simulink model "timedIzhikevichTest"  (R2020b)
settings: Solver=VariableStepAuto  StartTime=0.0  StopTime=5000  FixedStep=0.001  RelTol=1e-3
libraries: simulink x2, dspsigops x1
settings Model: PacingRate=0.071000  Creator=40129232  LastModifiedBy=adamalcorn
settings SolverCC: AlgebraicLoopSolver=LineSearch
settings DataIOCC: ReturnWorkspaceOutputs=off
settings OptimizationCC: LifeSpan=inf
settings DebuggingCC: SFExecutionAtInitializationDiag=none  ArithmeticOperatorsInVariantConditions=warning
settings SFSimCC: SimUseLocalCustomCode=off  CustomCodeUndefinedFunction=UseInterfaceOnly
settings RTWCC: RTWUseLocalCustomCode=off
settings CodeAppCC: StateflowObjectComments=on

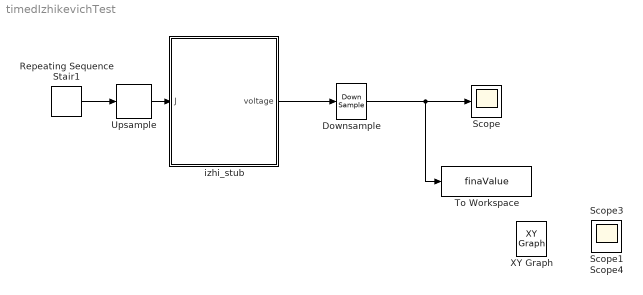
== system timedIzhikevichTest ==
  Downsample : DownSample  N=10  RateOptions=Allow multirate processing
  Repeating Sequence Stair1 : simulink/Sources/Repeating Sequence Stair  OutValues=[40.37, 52.35, 62.17, 70.19, 76.75].'  tsamp=10  OutMin=[]  OutMax=[]  OutDataTypeStr=double  OutputDataTypeScalingMode=double  OutDataType=fixdt(0,8)  ConRadixGroup=Best Precision: Vector-wise  OutScaling=2^-12
  Scope{,1,3..4} (4 alike) : Scope
  To Workspace : ToWorkspace  VariableName=finaValue  SaveFormat=Timeseries  SampleTime=-1
  Upsample : dspsigops/Upsample  N=10  phase=0  RateOptions=Allow multirate processing  ic=0  mode=Unused parameter value
  izhi_stub : Subsystem
  XY Graph : simulink/Sinks/XY Graph  IOType=viewer  xmin=-1  xmax=1  ymin=-1  ymax=1  st=-1
  wires:
  Repeating Sequence Stair1/1 -> Upsample/1
  Upsample/1 -> izhi_stub/1(J)
  Downsample/1 -> To Workspace/1, Scope/1
  izhi_stub/1(voltage) -> Downsample/1

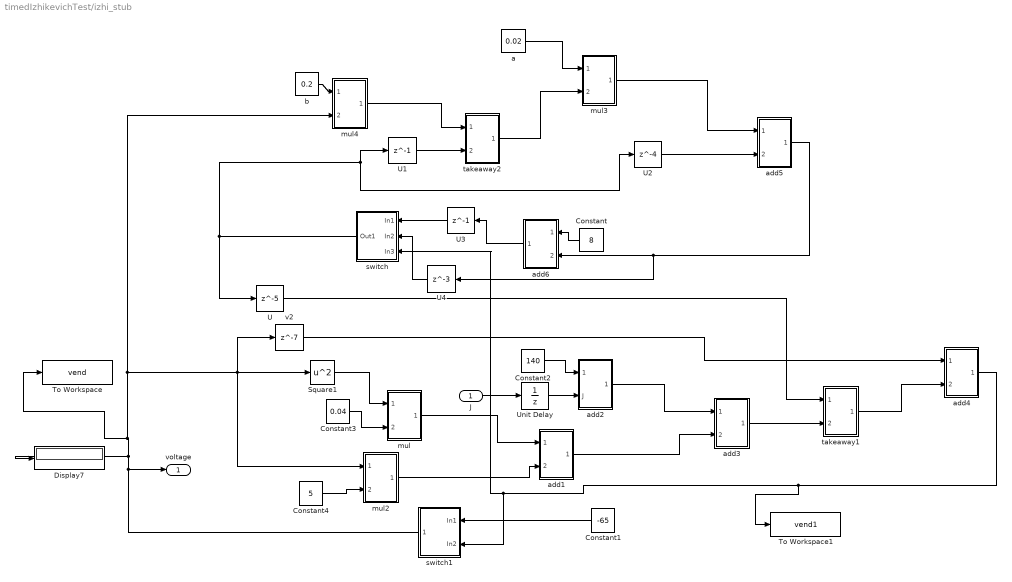
== system timedIzhikevichTest/izhi_stub ==
  J : Inport
  Constant : Constant  Value=8
  Constant1 : Constant  Value=-65
  Constant2 : Constant  Value=140
  Constant3 : Constant  Value=0.04
  Constant4 : Constant  Value=5
  Display7 : Display
  Square1 : Math  Operator=square  SaturateOnIntegerOverflow=on
  To Workspace : ToWorkspace  VariableName=vend  SaveFormat=Timeseries  SampleTime=-1
  To Workspace1 : ToWorkspace  VariableName=vend1  SaveFormat=Timeseries  SampleTime=-1
  U : Delay  DelayLength=5  InitialCondition=-65
  U1 : Delay  DelayLength=1  InitialCondition=0
  U2 : Delay  DelayLength=4  InitialCondition=0
  U3 : Delay  DelayLength=1  InitialCondition=0
  U4 : Delay  DelayLength=3  InitialCondition=0
  Unit Delay : UnitDelay  InitialCondition=-65  SampleTime=-1  HasFrameUpgradeWarning=on
  a : Constant  Value=0.02
  add1 : Subsystem
  add2 : Subsystem
  add3 : Subsystem
  add4 : Subsystem
  add5 : Subsystem
  add6 : Subsystem
  b : Constant  Value=0.2
  mul : Subsystem
  mul2 : Subsystem
  mul3 : Subsystem
  mul4 : Subsystem
  switch : Subsystem
  switch1 : Subsystem
  takeaway1 : Subsystem
  takeaway2 : Subsystem
  v2 : Delay  DelayLength=7  InitialCondition=-65
  voltage : Outport  VectorParamsAs1DForOutWhenUnconnected=off
  wires:
  Square1/1 -> mul/1(In1)
  Constant3/1 -> mul/2(In2)
  Constant4/1 -> mul2/2(In2)
  Constant2/1 -> add2/1(In1)
  Constant/1 -> add6/1(In1)
  a/1 -> mul3/1(In1)
  b/1 -> mul4/1(In1)
  Constant1/1 -> switch1/1(In1)
  add6/1(Out1) -> U3/1
  v2/1 -> add4/1(voltage)
  mul2/1(Out1) -> add1/2(In2)
  mul/1(Out1) -> add1/1(In1)
  add1/1(Out1) -> add3/2(In2)
  add3/1(Out1) -> takeaway1/2(In2)
  takeaway1/1(Out1) -> add4/2(In2)
  U/1 -> takeaway1/1(In1)
  add4/1(Out1) -> To Workspace1/1, switch/3(In3), switch1/2(In2)
  mul4/1(Out1) -> takeaway2/1(In1)
  switch/1(Out1) -> U1/1, U2/1, U/1
  U1/1 -> takeaway2/2(In2)
  U2/1 -> add5/2(In2)
  takeaway2/1(Out1) -> mul3/2(In2)
  mul3/1(Out1) -> add5/1(In1)
  add5/1(Out1) -> add6/2(In2), U4/1
  U4/1 -> switch/2(In2)
  U3/1 -> switch/1(In1)
  switch1/1(voltage) -> To Workspace/1, Square1/1, mul2/1(voltage), v2/1, mul4/2(voltage), Display7/1, voltage/1
  add2/1(Out1) -> add3/1(In1)
  J/1 -> Unit Delay/1
  Unit Delay/1 -> add2/2(J)

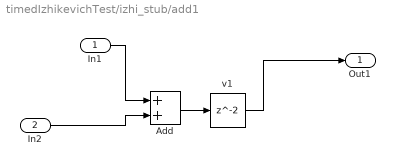
== system timedIzhikevichTest/izhi_stub/add1 ==
  In1 : Inport
  In2 : Inport  Port=2
  Add : Sum
  v1 : Delay  InitialCondition=-65
  Out1 : Outport
  wires:
  In2/1 -> Add/2
  In1/1 -> Add/1
  Add/1 -> v1/1
  v1/1 -> Out1/1

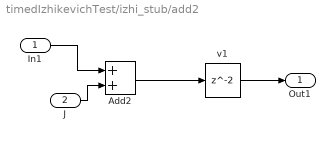
== system timedIzhikevichTest/izhi_stub/add2 ==
  In1 : Inport
  J : Inport  Port=2
  Add2 : Sum
  v1 : Delay  InitialCondition=-65
  Out1 : Outport
  wires:
  J/1 -> Add2/2
  In1/1 -> Add2/1
  Add2/1 -> v1/1
  v1/1 -> Out1/1

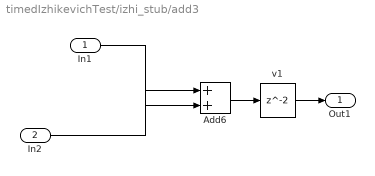
== system timedIzhikevichTest/izhi_stub/add3 ==
  In1 : Inport
  In2 : Inport  Port=2
  Add6 : Sum
  v1 : Delay  InitialCondition=-65
  Out1 : Outport
  wires:
  In2/1 -> Add6/1
  In1/1 -> Add6/2
  Add6/1 -> v1/1
  v1/1 -> Out1/1

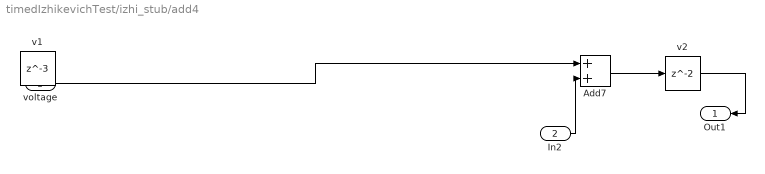
== system timedIzhikevichTest/izhi_stub/add4 ==
  voltage : Inport
  In2 : Inport  Port=2
  Add7 : Sum
  v1 : Delay  DelayLength=3  InitialCondition=0
  v2 : Delay  InitialCondition=-65
  Out1 : Outport
  wires:
  voltage/1 -> Add7/1
  In2/1 -> Add7/2
  Add7/1 -> v2/1
  v2/1 -> Out1/1

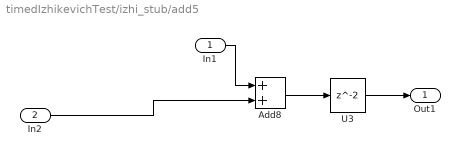
== system timedIzhikevichTest/izhi_stub/add5 ==
  In1 : Inport
  In2 : Inport  Port=2
  Add8 : Sum
  U3 : Delay  InitialCondition=0
  Out1 : Outport
  wires:
  In2/1 -> Add8/2
  In1/1 -> Add8/1
  Add8/1 -> U3/1
  U3/1 -> Out1/1

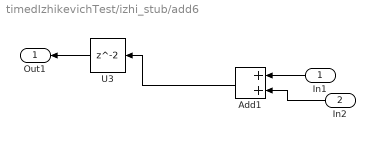
== system timedIzhikevichTest/izhi_stub/add6 ==
  In1 : Inport
  In2 : Inport  Port=2
  Add1 : Sum
  U3 : Delay  InitialCondition=0
  Out1 : Outport
  wires:
  In1/1 -> Add1/1
  In2/1 -> Add1/2
  Add1/1 -> U3/1
  U3/1 -> Out1/1

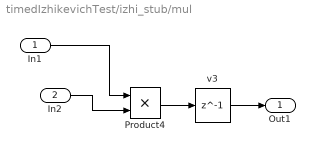
== system timedIzhikevichTest/izhi_stub/mul ==
  In1 : Inport
  In2 : Inport  Port=2
  Product4 : Product
  v3 : Delay  DelayLength=1  InitialCondition=-65
  Out1 : Outport
  wires:
  In2/1 -> Product4/2
  In1/1 -> Product4/1
  Product4/1 -> v3/1
  v3/1 -> Out1/1

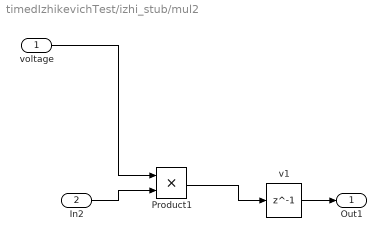
== system timedIzhikevichTest/izhi_stub/mul2 ==
  voltage : Inport
  In2 : Inport  Port=2
  Product1 : Product
  v1 : Delay  DelayLength=1  InitialCondition=-65
  Out1 : Outport
  wires:
  In2/1 -> Product1/2
  voltage/1 -> Product1/1
  Product1/1 -> v1/1
  v1/1 -> Out1/1

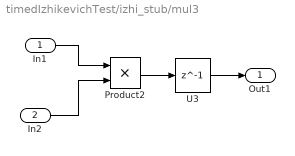
== system timedIzhikevichTest/izhi_stub/mul3 ==
  In1 : Inport
  In2 : Inport  Port=2
  Product2 : Product
  U3 : Delay  DelayLength=1  InitialCondition=0
  Out1 : Outport
  wires:
  In2/1 -> Product2/2
  In1/1 -> Product2/1
  Product2/1 -> U3/1
  U3/1 -> Out1/1

== system timedIzhikevichTest/izhi_stub/mul4 ==
  In1 : Inport
  voltage : Inport  Port=2
  Product3 : Product
  U2 : Delay  DelayLength=1  InitialCondition=0
  Out1 : Outport
  wires:
  voltage/1 -> Product3/2
  In1/1 -> Product3/1
  Product3/1 -> U2/1
  U2/1 -> Out1/1

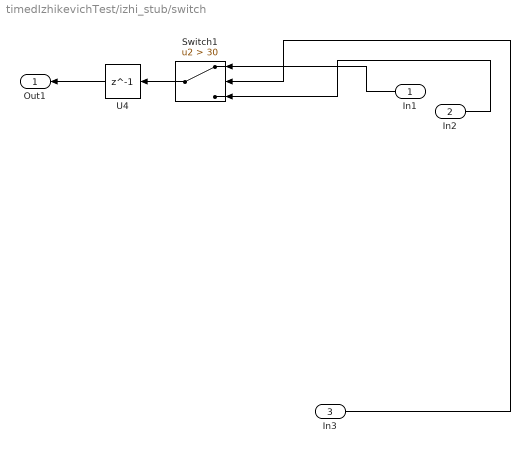
== system timedIzhikevichTest/izhi_stub/switch ==
  In1 : Inport
  In2 : Inport  Port=2
  In3 : Inport  Port=3
  Switch1 : Switch  Criteria=u2 > Threshold  Threshold=30
  U4 : Delay  DelayLength=1  InitialCondition=0
  Out1 : Outport
  wires:
  In1/1 -> Switch1/1
  In3/1 -> Switch1/2
  In2/1 -> Switch1/3
  Switch1/1 -> U4/1
  U4/1 -> Out1/1

== system timedIzhikevichTest/izhi_stub/switch1 ==
  In1 : Inport
  In2 : Inport  Port=2
  Switch : Switch  Criteria=u2 > Threshold  Threshold=30
  v1 : Delay  DelayLength=1  InitialCondition=-65
  voltage : Outport
  wires:
  In1/1 -> Switch/1
  In2/1 -> Switch/3, Switch/2
  Switch/1 -> v1/1
  v1/1 -> voltage/1

== system timedIzhikevichTest/izhi_stub/takeaway1 ==
  In1 : Inport
  In2 : Inport  Port=2
  Minus : Sum  Inputs=+-
  v1 : Delay  InitialCondition=-65
  Out1 : Outport
  wires:
  In2/1 -> Minus/1
  In1/1 -> Minus/2
  Minus/1 -> v1/1
  v1/1 -> Out1/1

== system timedIzhikevichTest/izhi_stub/takeaway2 ==
  In1 : Inport
  In2 : Inport  Port=2
  Minus2 : Sum  Inputs=+-
  U2 : Delay  InitialCondition=0
  Out1 : Outport
  wires:
  In2/1 -> Minus2/2
  In1/1 -> Minus2/1
  Minus2/1 -> U2/1
  U2/1 -> Out1/1
